simulink model "main"  (R2020b)
settings: Solver=ode23tb  StartTime=0.0  StopTime=20  FixedStep=0.0005  MaxStep=0.005  RelTol=1e-3  AbsTol=1e-3
StartFcn:
  | tic;
StopFcn:
  | Elapsed_Sim_Time = toc;
  | disp(['Elapsed Sim Time = ' num2str(Elapsed_Sim_Time)]);
model workspace (MATLAB code in the model file):
  | floor_l = 1.0900;
  | floor_d = 0.0100;
  | 
  | % PART
  | model_idx = 0;
  | model_dims = [0.06 0.06 0.06;
  |      0.02 0.05 0.07;
  |      0.04 0.04 0.10;
  |      0.05 0.05 0.05;
  |      0.10 0.08 0.08];
  | % distance between models on the conveyor belt
  | model_d = 0.12;
  | % distance to push models forwards in the -y dir (towards the box)
  | model_push = 0.2;
  | 
  | % BELT
  | belt_w = 0.1000;
  | belt_l = 1.2000;
  | belt_h = 0.0200;
  | belt_in_offset = [0 0.8000 0.0100];
  | 
  | container_belt_h = 0.02;
  | container_belt_l = 2.0;
  | container_belt_w = 0.2;
  | container_belt_offset = [-0.5050 0 -0.020];
  | 
  | belt_spd = 0.1;
  | 
  | % Model
  | cube_d = 0.06;
  | cube_z_off = belt_in_offset(3) + (container_belt_h / 2) + 0.001;
  | cube_z_offs = (model_dims(:,3) / 2) + cube_z_off;
  | 
  | % Container dimensions
  | % len, width, height are INTERNAL (Changed because most things were using internal anyway and it's 4am and we just need a working demo)
  | % Dimensions
  | container_len = 0.2;
  | container_width = 0.15;
  | container_height = 0.15;
  | container_thickness = 0.005;
  | 
  | 
  | % ????
  | cube_con_rsph = 0.003;
  | 
  | cube_con_k = 1000000;
  | cube_con_b = 1000;
  | 
  | finger_con_x = 0.01;
  | finger_con_y = 0.01;
  | finger_con_z = 5e-4;
  | finger_con_rsph = 5.0000e-04;
  | finger_con_muk = 0.05;
  | finger_con_mus = 0.07;
  | finger_con_vth = 1e-3;
  | 
  | finger_l = 0.4;
  | finger_w = 0.03;
  | finger_t = 0.01;
undefined symbols (not defined in the file): Bottom, Extr_Data_LinkHoles, Part1, Part2, Part3, Part4, Part5, point1, point2, point3, Side1, Side2, Side3, Side4, X, Y, Z
libraries: sm_lib x113, nesl_utility x35, Parts_Lib x10, Contact_Forces_Lib x6, sm_delta_robot_lib x1
(part 4 of 5)

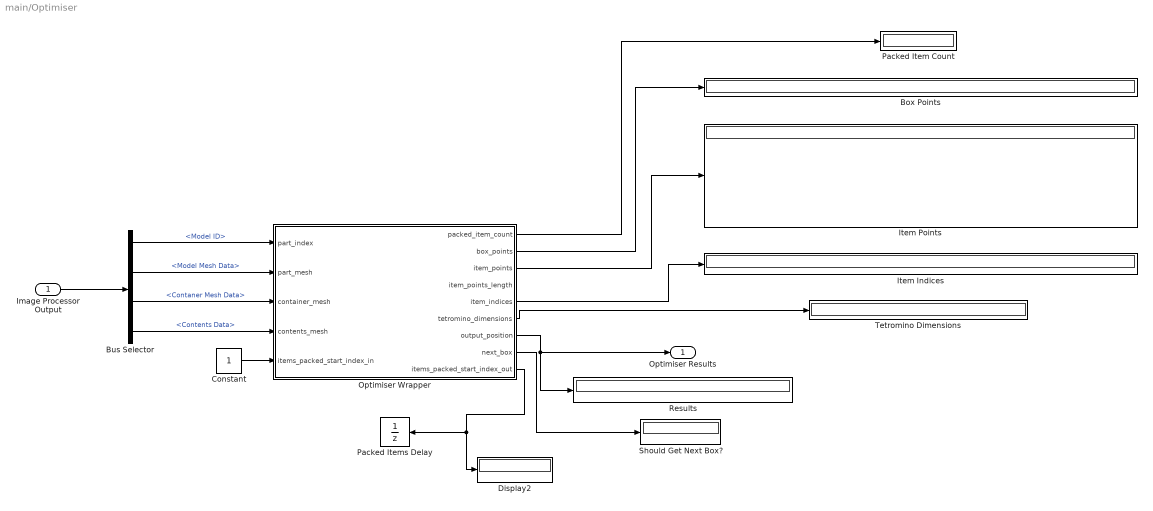
== system main/Optimiser ==
  Image Processor Output : Inport
  Box Points : Display
  Bus Selector : BusSelector  OutputSignals=Model ID,Model Mesh Data,Contaner Mesh Data,Contents Data
  Constant : Constant
  Display2 : Display
  Item Indices : Display
  Item Points : Display
  Optimiser Wrapper : MATLAB Function  TreatAsAtomicUnit=on
  Packed Item Count : Display
  Packed Items Delay : UnitDelay  InitialCondition=1  SampleTime=-1  HasFrameUpgradeWarning=on
  Results : Display
  Should Get Next Box? : Display
  Tetromino Dimensions : Display
  Optimiser Results : Outport
  wires:
  Optimiser Wrapper/8(next_box) -> Should Get Next Box?/1
  Optimiser Wrapper/9(items_packed_start_index_out) -> Packed Items Delay/1, Display2/1
  Optimiser Wrapper/2(box_points) -> Box Points/1
  Optimiser Wrapper/3(item_points) -> Item Points/1
  Optimiser Wrapper/5(item_indices) -> Item Indices/1
  Optimiser Wrapper/6(tetromino_dimensions) -> Tetromino Dimensions/1
  Image Processor Output/1 -> Bus Selector/1
  Bus Selector/1 -> Optimiser Wrapper/1(part_index)  "<Model ID>"
  Bus Selector/2 -> Optimiser Wrapper/2(part_mesh)  "<Model Mesh Data>"
  Bus Selector/3 -> Optimiser Wrapper/3(container_mesh)  "<Contaner Mesh Data>"
  Bus Selector/4 -> Optimiser Wrapper/4(contents_mesh)  "<Contents Data>"
  Optimiser Wrapper/1(packed_item_count) -> Packed Item Count/1
  Optimiser Wrapper/7(output_position) -> Optimiser Results/1, Results/1
  Constant/1 -> Optimiser Wrapper/5(items_packed_start_index_in)

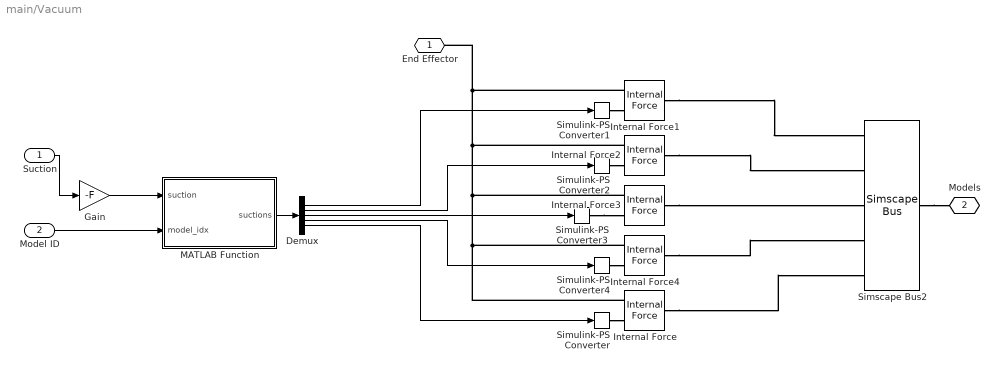
== system main/Vacuum ==
  Suction : Inport
  Model ID : Inport  Port=2
  Demux : Demux  Outputs=5
  Gain : Gain  Gain=-F
  Internal Force{,1..4} (5 alike) : sm_lib/Forces and Torques/Internal Force
      settings: SourceProductName=Multibody
  MATLAB Function : MATLAB Function  TreatAsAtomicUnit=on
  Simscape Bus2 : SimscapeBus  HierarchyStrings=Part1;Part2;Part3;Part4;Part5
  Simulink-PS Converter{,1..4} (5 alike) : nesl_utility/Simulink-PS Converter  PhysicalDomain=network_engine_domain  SubClassName=ps_input  LeftPortType=input  RightPortType=output  PseudoPeriodic=off  Frequencies=[]  NoiseDistribution=none  NoiseParameters=[]  Unit=N  AffineConversion=off  FilteringAndDerivatives=provide  SimscapeFilterOrder=1  InputFilterTimeConstant=0.001  UdotUserProvided=0
      settings: SourceProductName=Utilities
  End Effector : PMIOPort  Side=Right
  Models : PMIOPort  Port=2  Side=Right
  wires:
  Suction/1 -> Gain/1
  MATLAB Function/1(suctions) -> Demux/1
  Gain/1 -> MATLAB Function/1(suction)
  Demux/1 -> Simulink-PS Converter1/1
  Demux/2 -> Simulink-PS Converter2/1
  Demux/3 -> Simulink-PS Converter3/1
  Demux/4 -> Simulink-PS Converter4/1
  Demux/5 -> Simulink-PS Converter/1
  Model ID/1 -> MATLAB Function/2(model_idx)
  connections:
  Internal Force/RConn1 -- Simscape Bus2/LConn5
  Internal Force/LConn1 -- Internal Force4/LConn1 -- Internal Force3/LConn1 -- Internal Force2/LConn1 -- End Effector/RConn1 -- Internal Force1/LConn1
  Simulink-PS Converter/RConn1 -- Internal Force/LConn2
  Simscape Bus2/RConn1 -- Models/RConn1
  Simulink-PS Converter1/RConn1 -- Internal Force1/LConn2
  Simulink-PS Converter2/RConn1 -- Internal Force2/LConn2
  Simulink-PS Converter3/RConn1 -- Internal Force3/LConn2
  Simulink-PS Converter4/RConn1 -- Internal Force4/LConn2
  Internal Force4/RConn1 -- Simscape Bus2/LConn4
  Internal Force3/RConn1 -- Simscape Bus2/LConn3
  Internal Force2/RConn1 -- Simscape Bus2/LConn2
  Internal Force1/RConn1 -- Simscape Bus2/LConn1

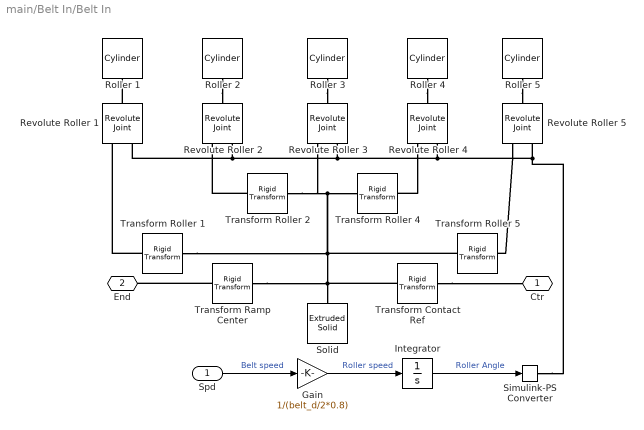
== system main/Belt In/Belt In ==
  Spd : Inport
  Gain : Gain  Gain=1/(belt_d/2*0.8)
  Integrator : Integrator
  Revolute Roller {1..5} (5 alike) : sm_lib/Joints/Revolute Joint  JointMode=Normal  SenseConstraintForce=off  SenseConstraintForceX=off  SenseConstraintForceY=off  SenseConstraintForceZ=off  SenseConstraintTorque=off  SenseConstraintTorqueX=off  SenseConstraintTorqueY=off  SenseConstraintTorqueZ=off  SenseTotalForce=off  SenseTotalForceX=off  SenseTotalForceY=off  SenseTotalForceZ=off  SenseTotalTorque=off  SenseTotalTorqueX=off  SenseTotalTorqueY=off  SenseTotalTorqueZ=off  CompositeWrenchDir=FollowerOnBase  CompositeWrenchFrame=BaseFrame  EquilibriumPosition=0  EquilibriumPositionUnits=deg  SpringStiffness=0  SpringStiffnessUnits=N*m/deg  DampingCoefficient=0  DampingCoefficientUnits=N*m/(deg/s)  TorqueActuationMode=ComputedTorque  MotionActuationMode=InputMotion  SensePosition=off  SenseVelocity=off  SenseAcceleration=off  SenseTorqueForce=off  SenseLowerLimitTorqueForce=off  SenseUpperLimitTorqueForce=off  LowerLimitSpecify=off  LowerLimitBound=-90  LowerLimitBoundUnits=deg  LowerLimitStiffness=1e4  LowerLimitStiffnessUnits=N*m/deg  LowerLimitDamping=10  LowerLimitDampingUnits=N*m/(deg/s)  LowerLimitTransitionRegionWidth=0.1  LowerLimitTransitionRegionWidthUnits=deg  UpperLimitSpecify=off  UpperLimitBound=90  UpperLimitBoundUnits=deg  UpperLimitStiffness=1e4  UpperLimitStiffnessUnits=N*m/deg  UpperLimitDamping=10  UpperLimitDampingUnits=N*m/(deg/s)  UpperLimitTransitionRegionWidth=0.1  UpperLimitTransitionRegionWidthUnits=deg  PositionTargetSpecify=off  PositionTargetPriority=High  PositionTargetValue=0  PositionTargetValueUnits=deg  VelocityTargetSpecify=off  VelocityTargetPriority=High  VelocityTargetValue=0  VelocityTargetValueUnits=deg/s
  Roller {1..5} (5 alike) : Parts_Lib/Cylinder  Tag=CustomStyle  cyl_radius=belt_d/2*0.8  cyl_length=belt_w  cyl_density=1000  cyl_color=custom  cyl_opacity=1  cyl_color_custom=roller_clr  mark_radius=[0.75 0.5]  mark_len_factor=1.01  mark_angle=60  mark_color=black  mark_opacity=1
  Simulink-PS Converter : nesl_utility/Simulink-PS Converter  PhysicalDomain=network_engine_domain  SubClassName=ps_input  LeftPortType=input  RightPortType=output  PseudoPeriodic=off  Frequencies=[]  NoiseDistribution=none  NoiseParameters=[]  Unit=1  AffineConversion=off  FilteringAndDerivatives=filter  SimscapeFilterOrder=2  InputFilterTimeConstant=0.005  UdotUserProvided=1
  Solid : sm_lib/Body Elements/Extruded Solid  GraphicAmbientColor=[0.15 0.15 0.15 1.0]  BasedOnType=Density  CenterOfMass=[0 0 0]  CenterOfMassUnits=m  GraphicDiffuseColor=[0.5 0.5 0.5]  ExportConvexHullGeometry=off  ExtrusionCrossSection=Extr_Data_LinkHoles(belt_l,belt_d,0.8*belt_d/2,5)  ExtrusionCrossSectionUnits=m  Density=1000  DensityUnits=kg/(m^3)  DoExposeReferenceFrame=on  GraphicEmissiveColor=[0.0 0.0 0.0 1.0]  ExportEntireGeometry=off  ExtrusionLength=belt_w  ExtrusionLengthUnits=m  ExtrusionType=General  SerializedFrames=<Frames/>  MarkerShape=Sphere  MarkerSize=10  GraphicType=FromGeometry  InertiaType=CalculateFromGeometry  Mass=1  MassUnits=kg  MomentsOfInertia=[1 1 1]  MomentsOfInertiaUnits=kg*m^2  PolygonNumSides=3  GraphicOpacity=1.0  PolygonOuterRadius=1  PolygonOuterRadiusUnits=m  ProductsOfInertia=[0 0 0]  ProductsOfInertiaUnits=kg*m^2  GraphicShininess=75  GraphicSpecularColor=[0.5 0.5 0.5 1.0]  GraphicVisPropType=SimpleVisualProperties
  Transform Contact Ref : sm_lib/Frames and Transforms/Rigid Transform  TranslationMethod=None  TranslationStandardOffset=3/2  TranslationLengthUnit=m  TranslationStandardAxis=+X  TranslationCartesianOffset=[0 0 0]  TranslationROffset=0  TranslationROffsetUnits=m  TranslationZOffset=0  TranslationZOffsetUnits=m  TranslationThetaOffset=0  TranslationThetaOffsetUnits=deg  RotationMethod=RotationSequence  RotationAngleUnits=deg  RotationStandardAxis=+Z  RotationAngle=0  RotationArbitraryAxis=[0 0 1]  FollAlignAxisA=+X  BaseAlignAxisA=+Y  FollAlignAxisB=+Y  BaseAlignAxisB=+Z  RotationSequenceAxes=FollowerAxes  RotationSequence=XYZ  RotationSequenceAngles=[-90 0 0]  RotationSequenceAnglesUnits=deg  RotationMatrix=[1 0 0; 0 1 0; 0 0 1]
  Transform Ramp Center : sm_lib/Frames and Transforms/Rigid Transform  TranslationMethod=StandardAxis  TranslationStandardOffset=belt_l/2  TranslationLengthUnit=m  TranslationStandardAxis=-X  TranslationCartesianOffset=[0 0 0]  TranslationROffset=0  TranslationROffsetUnits=m  TranslationZOffset=0  TranslationZOffsetUnits=m  TranslationThetaOffset=0  TranslationThetaOffsetUnits=deg  RotationMethod=None  RotationAngleUnits=deg  RotationStandardAxis=+Z  RotationAngle=0  RotationArbitraryAxis=[0 0 1]  FollAlignAxisA=+X  BaseAlignAxisA=+Y  FollAlignAxisB=+Y  BaseAlignAxisB=+Z  RotationSequenceAxes=FollowerAxes  RotationSequence=XYX  RotationSequenceAngles=[0 0 0]  RotationSequenceAnglesUnits=deg  RotationMatrix=[1 0 0; 0 1 0; 0 0 1]
  Transform Roller 1 : sm_lib/Frames and Transforms/Rigid Transform  TranslationMethod=StandardAxis  TranslationStandardOffset=belt_l/2  TranslationLengthUnit=m  TranslationStandardAxis=-X  TranslationCartesianOffset=[0 0 0]  TranslationROffset=0  TranslationROffsetUnits=m  TranslationZOffset=0  TranslationZOffsetUnits=m  TranslationThetaOffset=0  TranslationThetaOffsetUnits=deg  RotationMethod=None  RotationAngleUnits=deg  RotationStandardAxis=+Z  RotationAngle=0  RotationArbitraryAxis=[0 0 1]  FollAlignAxisA=+X  BaseAlignAxisA=+Y  FollAlignAxisB=+Y  BaseAlignAxisB=+Z  RotationSequenceAxes=FollowerAxes  RotationSequence=XYX  RotationSequenceAngles=[0 0 0]  RotationSequenceAnglesUnits=deg  RotationMatrix=[1 0 0; 0 1 0; 0 0 1]
  Transform Roller 2 : sm_lib/Frames and Transforms/Rigid Transform  TranslationMethod=StandardAxis  TranslationStandardOffset=belt_l/4  TranslationLengthUnit=m  TranslationStandardAxis=-X  TranslationCartesianOffset=[0 0 0]  TranslationROffset=0  TranslationROffsetUnits=m  TranslationZOffset=0  TranslationZOffsetUnits=m  TranslationThetaOffset=0  TranslationThetaOffsetUnits=deg  RotationMethod=None  RotationAngleUnits=deg  RotationStandardAxis=+Z  RotationAngle=0  RotationArbitraryAxis=[0 0 1]  FollAlignAxisA=+X  BaseAlignAxisA=+Y  FollAlignAxisB=+Y  BaseAlignAxisB=+Z  RotationSequenceAxes=FollowerAxes  RotationSequence=XYX  RotationSequenceAngles=[0 0 0]  RotationSequenceAnglesUnits=deg  RotationMatrix=[1 0 0; 0 1 0; 0 0 1]
  Transform Roller 4 : sm_lib/Frames and Transforms/Rigid Transform  TranslationMethod=StandardAxis  TranslationStandardOffset=belt_l/4  TranslationLengthUnit=m  TranslationStandardAxis=+X  TranslationCartesianOffset=[0 0 0]  TranslationROffset=0  TranslationROffsetUnits=m  TranslationZOffset=0  TranslationZOffsetUnits=m  TranslationThetaOffset=0  TranslationThetaOffsetUnits=deg  RotationMethod=None  RotationAngleUnits=deg  RotationStandardAxis=+Z  RotationAngle=0  RotationArbitraryAxis=[0 0 1]  FollAlignAxisA=+X  BaseAlignAxisA=+Y  FollAlignAxisB=+Y  BaseAlignAxisB=+Z  RotationSequenceAxes=FollowerAxes  RotationSequence=XYX  RotationSequenceAngles=[0 0 0]  RotationSequenceAnglesUnits=deg  RotationMatrix=[1 0 0; 0 1 0; 0 0 1]
  Transform Roller 5 : sm_lib/Frames and Transforms/Rigid Transform  TranslationMethod=StandardAxis  TranslationStandardOffset=belt_l/2  TranslationLengthUnit=m  TranslationStandardAxis=+X  TranslationCartesianOffset=[0 0 0]  TranslationROffset=0  TranslationROffsetUnits=m  TranslationZOffset=0  TranslationZOffsetUnits=m  TranslationThetaOffset=0  TranslationThetaOffsetUnits=deg  RotationMethod=None  RotationAngleUnits=deg  RotationStandardAxis=+Z  RotationAngle=0  RotationArbitraryAxis=[0 0 1]  FollAlignAxisA=+X  BaseAlignAxisA=+Y  FollAlignAxisB=+Y  BaseAlignAxisB=+Z  RotationSequenceAxes=FollowerAxes  RotationSequence=XYX  RotationSequenceAngles=[0 0 0]  RotationSequenceAnglesUnits=deg  RotationMatrix=[1 0 0; 0 1 0; 0 0 1]
  Ctr : PMIOPort  Side=Right
  End : PMIOPort  Port=2  Side=Left
  wires:
  Integrator/1 -> Simulink-PS Converter/1  "Roller Angle"
  Gain/1 -> Integrator/1  "Roller speed"
  Spd/1 -> Gain/1  "Belt speed"
  connections:
  Revolute Roller 5/LConn2 -- Revolute Roller 4/LConn2 -- Revolute Roller 3/LConn2 -- Revolute Roller 2/LConn2 -- Revolute Roller 1/LConn2 -- Simulink-PS Converter/RConn1
  Roller 5/LConn1 -- Revolute Roller 5/RConn1
  Roller 4/LConn1 -- Revolute Roller 4/RConn1
  Roller 3/LConn1 -- Revolute Roller 3/RConn1
  Roller 2/LConn1 -- Revolute Roller 2/RConn1
  Transform Roller 1/RConn1 -- Revolute Roller 1/LConn1
  Revolute Roller 5/LConn1 -- Transform Roller 5/RConn1
  Revolute Roller 4/LConn1 -- Transform Roller 4/RConn1
  Transform Roller 2/RConn1 -- Revolute Roller 2/LConn1
  Revolute Roller 1/RConn1 -- Roller 1/LConn1
  Transform Ramp Center/LConn1 -- End/RConn1
  Transform Contact Ref/RConn1 -- Transform Ramp Center/RConn1 -- Transform Roller 5/LConn1 -- Transform Roller 1/LConn1 -- Transform Roller 4/LConn1 -- Transform Roller 2/LConn1 -- Revolute Roller 3/LConn1 -- Solid/RConn1
  Transform Contact Ref/LConn1 -- Ctr/RConn1

== system main/Belt In/Create Bus Belt In1 ==
  On : Inport
  Belt Speed : Gain  Gain=belt_spd
  Bus Creator : BusCreator  Inputs=3
  Constant : Constant
  Constant1 : Constant  Value=0
  bus : Outport  VectorParamsAs1DForOutWhenUnconnected=off
  wires:
  Constant1/1 -> Bus Creator/3  "vy"
  On/1 -> Belt Speed/1
  Constant/1 -> Bus Creator/1  "Enable"
  Bus Creator/1 -> bus/1
  Belt Speed/1 -> Bus Creator/2  "vx"

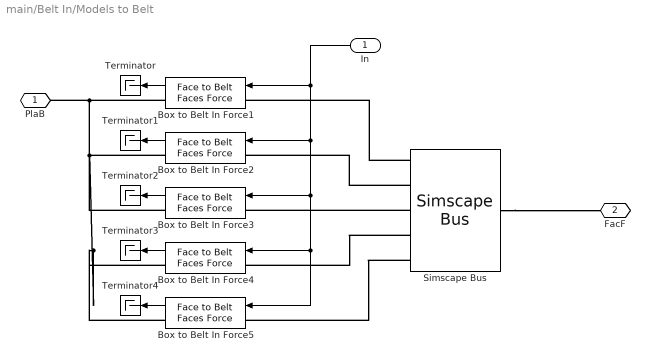
== system main/Belt In/Models to Belt ==
  In : Inport
  Box to Belt In Force1 : Contact_Forces_Lib/3D/Composite Forces/Face to Belt Faces Force  PlaB_x=belt_l  PlaB_y=belt_w  PlaB_z=belt_h/2  FacF_x=model_dims(1, 1)  FacF_y=model_dims(1, 2)  FacF_z=model_dims(1, 3)/2  FacF_rSph=cube_con_rsph  force_law_pla2pla=Linear  k_contact_pla2pla=stff  b_contact_pla2pla=dmp  pen_full_damp_F_pla2pla=1e-4  pen_exponent_pla2pla=1  friction_law_pla2pla=Stick-Slip Continuous  mu_kinetic_pla2pla=0.5  mu_static_pla2pla=0.7  v_thr_pla2pla=0.001  vis_on_pla2pla=off  vis_opc_en_box2box=0  vis_len_plaLz=0.0005  vis_clr=[0.9 0.2 0.2]  vis_opc=0.7
      settings: SourceProductName=Simscape Multibody Contact Forces Library
  Box to Belt In Force2 : Contact_Forces_Lib/3D/Composite Forces/Face to Belt Faces Force  PlaB_x=belt_l  PlaB_y=belt_w  PlaB_z=belt_h/2  FacF_x=model_dims(2, 1)  FacF_y=model_dims(2, 2)  FacF_z=model_dims(2, 3)/2  FacF_rSph=cube_con_rsph  force_law_pla2pla=Linear  k_contact_pla2pla=stff  b_contact_pla2pla=dmp  pen_full_damp_F_pla2pla=1e-4  pen_exponent_pla2pla=1  friction_law_pla2pla=Stick-Slip Continuous  mu_kinetic_pla2pla=0.5  mu_static_pla2pla=0.7  v_thr_pla2pla=0.001  vis_on_pla2pla=off  vis_opc_en_box2box=0  vis_len_plaLz=0.0005  vis_clr=[0.9 0.2 0.2]  vis_opc=0.7
      settings: SourceProductName=Simscape Multibody Contact Forces Library
  Box to Belt In Force3 : Contact_Forces_Lib/3D/Composite Forces/Face to Belt Faces Force  PlaB_x=belt_l  PlaB_y=belt_w  PlaB_z=belt_h/2  FacF_x=model_dims(3, 1)  FacF_y=model_dims(3, 2)  FacF_z=model_dims(3, 3)/2  FacF_rSph=cube_con_rsph  force_law_pla2pla=Linear  k_contact_pla2pla=stff  b_contact_pla2pla=dmp  pen_full_damp_F_pla2pla=1e-4  pen_exponent_pla2pla=1  friction_law_pla2pla=Stick-Slip Continuous  mu_kinetic_pla2pla=0.5  mu_static_pla2pla=0.7  v_thr_pla2pla=0.001  vis_on_pla2pla=off  vis_opc_en_box2box=0  vis_len_plaLz=0.0005  vis_clr=[0.9 0.2 0.2]  vis_opc=0.7
      settings: SourceProductName=Simscape Multibody Contact Forces Library
  Box to Belt In Force4 : Contact_Forces_Lib/3D/Composite Forces/Face to Belt Faces Force  PlaB_x=belt_l  PlaB_y=belt_w  PlaB_z=belt_h/2  FacF_x=model_dims(4, 1)  FacF_y=model_dims(4, 2)  FacF_z=model_dims(4, 3)/2  FacF_rSph=cube_con_rsph  force_law_pla2pla=Linear  k_contact_pla2pla=stff  b_contact_pla2pla=dmp  pen_full_damp_F_pla2pla=1e-4  pen_exponent_pla2pla=1  friction_law_pla2pla=Stick-Slip Continuous  mu_kinetic_pla2pla=0.5  mu_static_pla2pla=0.7  v_thr_pla2pla=0.001  vis_on_pla2pla=off  vis_opc_en_box2box=0  vis_len_plaLz=0.0005  vis_clr=[0.9 0.2 0.2]  vis_opc=0.7
      settings: SourceProductName=Simscape Multibody Contact Forces Library
  Box to Belt In Force5 : Contact_Forces_Lib/3D/Composite Forces/Face to Belt Faces Force  PlaB_x=belt_l  PlaB_y=belt_w  PlaB_z=belt_h/2  FacF_x=model_dims(5, 1)  FacF_y=model_dims(5, 2)  FacF_z=model_dims(5, 3)/2  FacF_rSph=cube_con_rsph  force_law_pla2pla=Linear  k_contact_pla2pla=stff  b_contact_pla2pla=dmp  pen_full_damp_F_pla2pla=1e-4  pen_exponent_pla2pla=1  friction_law_pla2pla=Stick-Slip Continuous  mu_kinetic_pla2pla=0.5  mu_static_pla2pla=0.7  v_thr_pla2pla=0.001  vis_on_pla2pla=off  vis_opc_en_box2box=0  vis_len_plaLz=0.0005  vis_clr=[0.9 0.2 0.2]  vis_opc=0.7
      settings: SourceProductName=Simscape Multibody Contact Forces Library
  Simscape Bus : SimscapeBus  HierarchyStrings=Part1;Part2;Part3;Part4;Part5
  Terminator{,1..4} (5 alike) : Terminator
  PlaB : PMIOPort  Side=Right
  FacF : PMIOPort  Port=2  Side=Left
  wires:
  Box to Belt In Force1/1 -> Terminator/1
  In/1 -> Box to Belt In Force1/1, Box to Belt In Force5/1, Box to Belt In Force4/1, Box to Belt In Force3/1, Box to Belt In Force2/1
  Box to Belt In Force2/1 -> Terminator1/1
  Box to Belt In Force5/1 -> Terminator4/1
  Box to Belt In Force4/1 -> Terminator3/1
  Box to Belt In Force3/1 -> Terminator2/1
  connections:
  Box to Belt In Force1/RConn1 -- Box to Belt In Force5/RConn1 -- Box to Belt In Force4/RConn1 -- Box to Belt In Force3/RConn1 -- Box to Belt In Force2/RConn1 -- PlaB/RConn1
  Simscape Bus/RConn1 -- FacF/RConn1
  Simscape Bus/LConn1 -- Box to Belt In Force1/LConn1
  Simscape Bus/LConn2 -- Box to Belt In Force2/LConn1
  Simscape Bus/LConn3 -- Box to Belt In Force3/LConn1
  Simscape Bus/LConn4 -- Box to Belt In Force4/LConn1
  Simscape Bus/LConn5 -- Box to Belt In Force5/LConn1

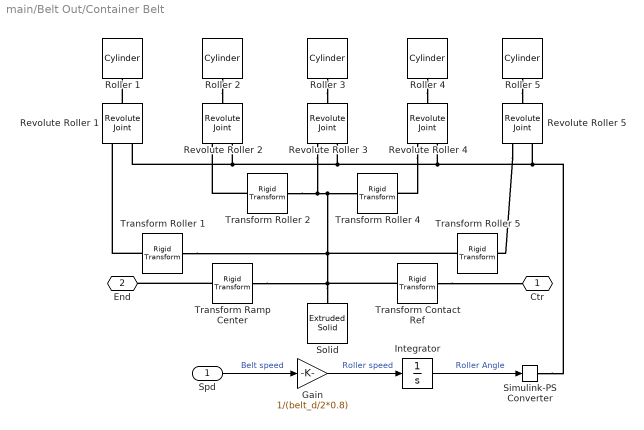
== system main/Belt Out/Container Belt ==
  Spd : Inport
  Gain : Gain  Gain=1/(belt_d/2*0.8)
  Integrator : Integrator
  Revolute Roller {1..5} (5 alike) : sm_lib/Joints/Revolute Joint  JointMode=Normal  SenseConstraintForce=off  SenseConstraintForceX=off  SenseConstraintForceY=off  SenseConstraintForceZ=off  SenseConstraintTorque=off  SenseConstraintTorqueX=off  SenseConstraintTorqueY=off  SenseConstraintTorqueZ=off  SenseTotalForce=off  SenseTotalForceX=off  SenseTotalForceY=off  SenseTotalForceZ=off  SenseTotalTorque=off  SenseTotalTorqueX=off  SenseTotalTorqueY=off  SenseTotalTorqueZ=off  CompositeWrenchDir=FollowerOnBase  CompositeWrenchFrame=BaseFrame  EquilibriumPosition=0  EquilibriumPositionUnits=deg  SpringStiffness=0  SpringStiffnessUnits=N*m/deg  DampingCoefficient=0  DampingCoefficientUnits=N*m/(deg/s)  TorqueActuationMode=ComputedTorque  MotionActuationMode=InputMotion  SensePosition=off  SenseVelocity=off  SenseAcceleration=off  SenseTorqueForce=off  SenseLowerLimitTorqueForce=off  SenseUpperLimitTorqueForce=off  LowerLimitSpecify=off  LowerLimitBound=-90  LowerLimitBoundUnits=deg  LowerLimitStiffness=1e4  LowerLimitStiffnessUnits=N*m/deg  LowerLimitDamping=10  LowerLimitDampingUnits=N*m/(deg/s)  LowerLimitTransitionRegionWidth=0.1  LowerLimitTransitionRegionWidthUnits=deg  UpperLimitSpecify=off  UpperLimitBound=90  UpperLimitBoundUnits=deg  UpperLimitStiffness=1e4  UpperLimitStiffnessUnits=N*m/deg  UpperLimitDamping=10  UpperLimitDampingUnits=N*m/(deg/s)  UpperLimitTransitionRegionWidth=0.1  UpperLimitTransitionRegionWidthUnits=deg  PositionTargetSpecify=off  PositionTargetPriority=High  PositionTargetValue=0  PositionTargetValueUnits=deg  VelocityTargetSpecify=off  VelocityTargetPriority=High  VelocityTargetValue=0  VelocityTargetValueUnits=deg/s
  Roller {1..5} (5 alike) : Parts_Lib/Cylinder  Tag=CustomStyle  cyl_radius=belt_d/2*0.8  cyl_length=belt_w  cyl_density=1000  cyl_color=custom  cyl_opacity=1  cyl_color_custom=roller_clr  mark_radius=[0.75 0.5]  mark_len_factor=1.01  mark_angle=60  mark_color=black  mark_opacity=1
  Simulink-PS Converter : nesl_utility/Simulink-PS Converter  PhysicalDomain=network_engine_domain  SubClassName=ps_input  LeftPortType=input  RightPortType=output  PseudoPeriodic=off  Frequencies=[]  NoiseDistribution=none  NoiseParameters=[]  Unit=1  AffineConversion=off  FilteringAndDerivatives=filter  SimscapeFilterOrder=2  InputFilterTimeConstant=0.005  UdotUserProvided=1
  Solid : sm_lib/Body Elements/Extruded Solid  GraphicAmbientColor=[0.15 0.15 0.15 1.0]  BasedOnType=Density  CenterOfMass=[0 0 0]  CenterOfMassUnits=m  GraphicDiffuseColor=[0.5 0.5 0.5]  ExportConvexHullGeometry=off  ExtrusionCrossSection=Extr_Data_LinkHoles(belt_l,belt_d,0.8*belt_d/2,5)  ExtrusionCrossSectionUnits=m  Density=1000  DensityUnits=kg/(m^3)  DoExposeReferenceFrame=on  GraphicEmissiveColor=[0.0 0.0 0.0 1.0]  ExportEntireGeometry=off  ExtrusionLength=belt_w  ExtrusionLengthUnits=m  ExtrusionType=General  SerializedFrames=<Frames/>  MarkerShape=Sphere  MarkerSize=10  GraphicType=FromGeometry  InertiaType=CalculateFromGeometry  Mass=1  MassUnits=kg  MomentsOfInertia=[1 1 1]  MomentsOfInertiaUnits=kg*m^2  PolygonNumSides=3  GraphicOpacity=1.0  PolygonOuterRadius=1  PolygonOuterRadiusUnits=m  ProductsOfInertia=[0 0 0]  ProductsOfInertiaUnits=kg*m^2  GraphicShininess=75  GraphicSpecularColor=[0.5 0.5 0.5 1.0]  GraphicVisPropType=SimpleVisualProperties
  Transform Contact Ref : sm_lib/Frames and Transforms/Rigid Transform  TranslationMethod=None  TranslationStandardOffset=3/2  TranslationLengthUnit=m  TranslationStandardAxis=+X  TranslationCartesianOffset=[0 0 0]  TranslationROffset=0  TranslationROffsetUnits=m  TranslationZOffset=0  TranslationZOffsetUnits=m  TranslationThetaOffset=0  TranslationThetaOffsetUnits=deg  RotationMethod=RotationSequence  RotationAngleUnits=deg  RotationStandardAxis=+Z  RotationAngle=0  RotationArbitraryAxis=[0 0 1]  FollAlignAxisA=+X  BaseAlignAxisA=+Y  FollAlignAxisB=+Y  BaseAlignAxisB=+Z  RotationSequenceAxes=FollowerAxes  RotationSequence=XYZ  RotationSequenceAngles=[-90 0 0]  RotationSequenceAnglesUnits=deg  RotationMatrix=[1 0 0; 0 1 0; 0 0 1]
  Transform Ramp Center : sm_lib/Frames and Transforms/Rigid Transform  TranslationMethod=StandardAxis  TranslationStandardOffset=belt_l/2  TranslationLengthUnit=m  TranslationStandardAxis=-X  TranslationCartesianOffset=[0 0 0]  TranslationROffset=0  TranslationROffsetUnits=m  TranslationZOffset=0  TranslationZOffsetUnits=m  TranslationThetaOffset=0  TranslationThetaOffsetUnits=deg  RotationMethod=None  RotationAngleUnits=deg  RotationStandardAxis=+Z  RotationAngle=0  RotationArbitraryAxis=[0 0 1]  FollAlignAxisA=+X  BaseAlignAxisA=+Y  FollAlignAxisB=+Y  BaseAlignAxisB=+Z  RotationSequenceAxes=FollowerAxes  RotationSequence=XYX  RotationSequenceAngles=[0 0 0]  RotationSequenceAnglesUnits=deg  RotationMatrix=[1 0 0; 0 1 0; 0 0 1]
  Transform Roller 1 : sm_lib/Frames and Transforms/Rigid Transform  TranslationMethod=StandardAxis  TranslationStandardOffset=belt_l/2  TranslationLengthUnit=m  TranslationStandardAxis=-X  TranslationCartesianOffset=[0 0 0]  TranslationROffset=0  TranslationROffsetUnits=m  TranslationZOffset=0  TranslationZOffsetUnits=m  TranslationThetaOffset=0  TranslationThetaOffsetUnits=deg  RotationMethod=None  RotationAngleUnits=deg  RotationStandardAxis=+Z  RotationAngle=0  RotationArbitraryAxis=[0 0 1]  FollAlignAxisA=+X  BaseAlignAxisA=+Y  FollAlignAxisB=+Y  BaseAlignAxisB=+Z  RotationSequenceAxes=FollowerAxes  RotationSequence=XYX  RotationSequenceAngles=[0 0 0]  RotationSequenceAnglesUnits=deg  RotationMatrix=[1 0 0; 0 1 0; 0 0 1]
  Transform Roller 2 : sm_lib/Frames and Transforms/Rigid Transform  TranslationMethod=StandardAxis  TranslationStandardOffset=belt_l/4  TranslationLengthUnit=m  TranslationStandardAxis=-X  TranslationCartesianOffset=[0 0 0]  TranslationROffset=0  TranslationROffsetUnits=m  TranslationZOffset=0  TranslationZOffsetUnits=m  TranslationThetaOffset=0  TranslationThetaOffsetUnits=deg  RotationMethod=None  RotationAngleUnits=deg  RotationStandardAxis=+Z  RotationAngle=0  RotationArbitraryAxis=[0 0 1]  FollAlignAxisA=+X  BaseAlignAxisA=+Y  FollAlignAxisB=+Y  BaseAlignAxisB=+Z  RotationSequenceAxes=FollowerAxes  RotationSequence=XYX  RotationSequenceAngles=[0 0 0]  RotationSequenceAnglesUnits=deg  RotationMatrix=[1 0 0; 0 1 0; 0 0 1]
  Transform Roller 4 : sm_lib/Frames and Transforms/Rigid Transform  TranslationMethod=StandardAxis  TranslationStandardOffset=belt_l/4  TranslationLengthUnit=m  TranslationStandardAxis=+X  TranslationCartesianOffset=[0 0 0]  TranslationROffset=0  TranslationROffsetUnits=m  TranslationZOffset=0  TranslationZOffsetUnits=m  TranslationThetaOffset=0  TranslationThetaOffsetUnits=deg  RotationMethod=None  RotationAngleUnits=deg  RotationStandardAxis=+Z  RotationAngle=0  RotationArbitraryAxis=[0 0 1]  FollAlignAxisA=+X  BaseAlignAxisA=+Y  FollAlignAxisB=+Y  BaseAlignAxisB=+Z  RotationSequenceAxes=FollowerAxes  RotationSequence=XYX  RotationSequenceAngles=[0 0 0]  RotationSequenceAnglesUnits=deg  RotationMatrix=[1 0 0; 0 1 0; 0 0 1]
  Transform Roller 5 : sm_lib/Frames and Transforms/Rigid Transform  TranslationMethod=StandardAxis  TranslationStandardOffset=belt_l/2  TranslationLengthUnit=m  TranslationStandardAxis=+X  TranslationCartesianOffset=[0 0 0]  TranslationROffset=0  TranslationROffsetUnits=m  TranslationZOffset=0  TranslationZOffsetUnits=m  TranslationThetaOffset=0  TranslationThetaOffsetUnits=deg  RotationMethod=None  RotationAngleUnits=deg  RotationStandardAxis=+Z  RotationAngle=0  RotationArbitraryAxis=[0 0 1]  FollAlignAxisA=+X  BaseAlignAxisA=+Y  FollAlignAxisB=+Y  BaseAlignAxisB=+Z  RotationSequenceAxes=FollowerAxes  RotationSequence=XYX  RotationSequenceAngles=[0 0 0]  RotationSequenceAnglesUnits=deg  RotationMatrix=[1 0 0; 0 1 0; 0 0 1]
  Ctr : PMIOPort  Side=Right
  End : PMIOPort  Port=2  Side=Left
  wires:
  Spd/1 -> Gain/1  "Belt speed"
  Gain/1 -> Integrator/1  "Roller speed"
  Integrator/1 -> Simulink-PS Converter/1  "Roller Angle"
  connections:
  Transform Contact Ref/LConn1 -- Ctr/RConn1
  Solid/RConn1 -- Revolute Roller 3/LConn1 -- Transform Roller 2/LConn1 -- Transform Roller 4/LConn1 -- Transform Roller 1/LConn1 -- Transform Roller 5/LConn1 -- Transform Ramp Center/RConn1 -- Transform Contact Ref/RConn1
  Transform Ramp Center/LConn1 -- End/RConn1
  Revolute Roller 1/RConn1 -- Roller 1/LConn1
  Transform Roller 2/RConn1 -- Revolute Roller 2/LConn1
  Revolute Roller 4/LConn1 -- Transform Roller 4/RConn1
  Revolute Roller 5/LConn1 -- Transform Roller 5/RConn1
  Transform Roller 1/RConn1 -- Revolute Roller 1/LConn1
  Roller 2/LConn1 -- Revolute Roller 2/RConn1
  Roller 3/LConn1 -- Revolute Roller 3/RConn1
  Roller 4/LConn1 -- Revolute Roller 4/RConn1
  Roller 5/LConn1 -- Revolute Roller 5/RConn1
  Simulink-PS Converter/RConn1 -- Revolute Roller 1/LConn2 -- Revolute Roller 2/LConn2 -- Revolute Roller 3/LConn2 -- Revolute Roller 4/LConn2 -- Revolute Roller 5/LConn2

== system main/Belt Out/Create Bus Belt Out ==
  On : Inport
  Belt Speed : Gain  Gain=belt_spd
  Bus Creator1 : BusCreator  Inputs=3
  Constant2 : Constant  Value=0
  Constant3 : Constant
  bus : Outport  VectorParamsAs1DForOutWhenUnconnected=off
  wires:
  On/1 -> Belt Speed/1
  Constant2/1 -> Bus Creator1/3  "vy"
  Bus Creator1/1 -> bus/1
  Constant3/1 -> Bus Creator1/1  "Enable"
  Belt Speed/1 -> Bus Creator1/2  "vx"

== system main/Contacts Models Container/Contacts Model-Container1 ==
  Simscape Bus : SimscapeBus  HierarchyStrings=Side1;Side2;Side3;Side4;Bottom
  Spatial Contact Force{1..3,7} (4 alike) : sm_lib/Forces and Torques/Spatial Contact Force  CoefficientOfDynamicFriction=muk  CoefficientOfStaticFriction=mus  NormalDamping=b  NormalDampingUnits=N/(m/s)  NormalStiffness=k  NormalStiffnessUnits=N/m  FrictionalCriticalVelocity=1e-3  FrictionalCriticalVelocityUnits=m/s  ZeroCrossDetectContactStartAndEnd=off  SenseFrictionalForceMagnitude=off  SenseNormalForceMagnitude=off  SenseSeparationDistance=off  NormalTransitionRegionWidth=1e-4  NormalTransitionRegionWidthUnits=m  FrictionType=SmoothStickSlip
      settings: SourceProductName=Multibody
  Spatial Contact Force4 : sm_lib/Forces and Torques/Spatial Contact Force  CoefficientOfDynamicFriction=muk  CoefficientOfStaticFriction=mus  NormalDamping=b  NormalDampingUnits=N/(m/s)  NormalStiffness=k  NormalStiffnessUnits=N/m  FrictionalCriticalVelocity=1e-3  FrictionalCriticalVelocityUnits=m/s  ZeroCrossDetectContactStartAndEnd=on  SenseFrictionalForceMagnitude=off  SenseNormalForceMagnitude=off  SenseSeparationDistance=off  NormalTransitionRegionWidth=1e-5  NormalTransitionRegionWidthUnits=m  FrictionType=SmoothStickSlip
      settings: SourceProductName=Multibody
  Container : PMIOPort  Side=Left
  Part : PMIOPort  Port=2  Side=Right
  connections:
  Spatial Contact Force4/RConn1 -- Spatial Contact Force3/RConn1 -- Part/RConn1 -- Spatial Contact Force2/RConn1 -- Spatial Contact Force1/RConn1 -- Spatial Contact Force7/RConn1
  Simscape Bus/RConn1 -- Container/RConn1
  Simscape Bus/LConn1 -- Spatial Contact Force7/LConn1
  Simscape Bus/LConn2 -- Spatial Contact Force1/LConn1
  Simscape Bus/LConn3 -- Spatial Contact Force2/LConn1
  Simscape Bus/LConn4 -- Spatial Contact Force3/LConn1
  Simscape Bus/LConn5 -- Spatial Contact Force4/LConn1

== system main/Contacts Models Container/Contacts Model-Container2 ==
  Simscape Bus : SimscapeBus  HierarchyStrings=Side1;Side2;Side3;Side4;Bottom
  Spatial Contact Force{1..3,7} (4 alike) : sm_lib/Forces and Torques/Spatial Contact Force  CoefficientOfDynamicFriction=muk  CoefficientOfStaticFriction=mus  NormalDamping=b  NormalDampingUnits=N/(m/s)  NormalStiffness=k  NormalStiffnessUnits=N/m  FrictionalCriticalVelocity=1e-3  FrictionalCriticalVelocityUnits=m/s  ZeroCrossDetectContactStartAndEnd=off  SenseFrictionalForceMagnitude=off  SenseNormalForceMagnitude=off  SenseSeparationDistance=off  NormalTransitionRegionWidth=1e-4  NormalTransitionRegionWidthUnits=m  FrictionType=SmoothStickSlip
      settings: SourceProductName=Multibody
  Spatial Contact Force4 : sm_lib/Forces and Torques/Spatial Contact Force  CoefficientOfDynamicFriction=muk  CoefficientOfStaticFriction=mus  NormalDamping=b  NormalDampingUnits=N/(m/s)  NormalStiffness=k  NormalStiffnessUnits=N/m  FrictionalCriticalVelocity=1e-3  FrictionalCriticalVelocityUnits=m/s  ZeroCrossDetectContactStartAndEnd=on  SenseFrictionalForceMagnitude=off  SenseNormalForceMagnitude=off  SenseSeparationDistance=off  NormalTransitionRegionWidth=1e-5  NormalTransitionRegionWidthUnits=m  FrictionType=SmoothStickSlip
      settings: SourceProductName=Multibody
  Container : PMIOPort  Side=Left
  Part : PMIOPort  Port=2  Side=Right
  connections:
  Spatial Contact Force4/RConn1 -- Spatial Contact Force3/RConn1 -- Part/RConn1 -- Spatial Contact Force2/RConn1 -- Spatial Contact Force1/RConn1 -- Spatial Contact Force7/RConn1
  Simscape Bus/RConn1 -- Container/RConn1
  Simscape Bus/LConn1 -- Spatial Contact Force7/LConn1
  Simscape Bus/LConn2 -- Spatial Contact Force1/LConn1
  Simscape Bus/LConn3 -- Spatial Contact Force2/LConn1
  Simscape Bus/LConn4 -- Spatial Contact Force3/LConn1
  Simscape Bus/LConn5 -- Spatial Contact Force4/LConn1

== system main/Contacts Models Container/Contacts Model-Container3 ==
  Simscape Bus : SimscapeBus  HierarchyStrings=Side1;Side2;Side3;Side4;Bottom
  Spatial Contact Force{1..3,7} (4 alike) : sm_lib/Forces and Torques/Spatial Contact Force  CoefficientOfDynamicFriction=muk  CoefficientOfStaticFriction=mus  NormalDamping=b  NormalDampingUnits=N/(m/s)  NormalStiffness=k  NormalStiffnessUnits=N/m  FrictionalCriticalVelocity=1e-3  FrictionalCriticalVelocityUnits=m/s  ZeroCrossDetectContactStartAndEnd=off  SenseFrictionalForceMagnitude=off  SenseNormalForceMagnitude=off  SenseSeparationDistance=off  NormalTransitionRegionWidth=1e-4  NormalTransitionRegionWidthUnits=m  FrictionType=SmoothStickSlip
      settings: SourceProductName=Multibody
  Spatial Contact Force4 : sm_lib/Forces and Torques/Spatial Contact Force  CoefficientOfDynamicFriction=muk  CoefficientOfStaticFriction=mus  NormalDamping=b  NormalDampingUnits=N/(m/s)  NormalStiffness=k  NormalStiffnessUnits=N/m  FrictionalCriticalVelocity=1e-3  FrictionalCriticalVelocityUnits=m/s  ZeroCrossDetectContactStartAndEnd=on  SenseFrictionalForceMagnitude=off  SenseNormalForceMagnitude=off  SenseSeparationDistance=off  NormalTransitionRegionWidth=1e-5  NormalTransitionRegionWidthUnits=m  FrictionType=SmoothStickSlip
      settings: SourceProductName=Multibody
  Container : PMIOPort  Side=Left
  Part : PMIOPort  Port=2  Side=Right
  connections:
  Spatial Contact Force4/RConn1 -- Spatial Contact Force3/RConn1 -- Part/RConn1 -- Spatial Contact Force2/RConn1 -- Spatial Contact Force1/RConn1 -- Spatial Contact Force7/RConn1
  Simscape Bus/RConn1 -- Container/RConn1
  Simscape Bus/LConn1 -- Spatial Contact Force7/LConn1
  Simscape Bus/LConn2 -- Spatial Contact Force1/LConn1
  Simscape Bus/LConn3 -- Spatial Contact Force2/LConn1
  Simscape Bus/LConn4 -- Spatial Contact Force3/LConn1
  Simscape Bus/LConn5 -- Spatial Contact Force4/LConn1

== system main/Contacts Models Container/Contacts Model-Container4 ==
  Simscape Bus : SimscapeBus  HierarchyStrings=Side1;Side2;Side3;Side4;Bottom
  Spatial Contact Force{1..3,7} (4 alike) : sm_lib/Forces and Torques/Spatial Contact Force  CoefficientOfDynamicFriction=muk  CoefficientOfStaticFriction=mus  NormalDamping=b  NormalDampingUnits=N/(m/s)  NormalStiffness=k  NormalStiffnessUnits=N/m  FrictionalCriticalVelocity=1e-3  FrictionalCriticalVelocityUnits=m/s  ZeroCrossDetectContactStartAndEnd=off  SenseFrictionalForceMagnitude=off  SenseNormalForceMagnitude=off  SenseSeparationDistance=off  NormalTransitionRegionWidth=1e-4  NormalTransitionRegionWidthUnits=m  FrictionType=SmoothStickSlip
      settings: SourceProductName=Multibody
  Spatial Contact Force4 : sm_lib/Forces and Torques/Spatial Contact Force  CoefficientOfDynamicFriction=muk  CoefficientOfStaticFriction=mus  NormalDamping=b  NormalDampingUnits=N/(m/s)  NormalStiffness=k  NormalStiffnessUnits=N/m  FrictionalCriticalVelocity=1e-3  FrictionalCriticalVelocityUnits=m/s  ZeroCrossDetectContactStartAndEnd=on  SenseFrictionalForceMagnitude=off  SenseNormalForceMagnitude=off  SenseSeparationDistance=off  NormalTransitionRegionWidth=1e-5  NormalTransitionRegionWidthUnits=m  FrictionType=SmoothStickSlip
      settings: SourceProductName=Multibody
  Container : PMIOPort  Side=Left
  Part : PMIOPort  Port=2  Side=Right
  connections:
  Spatial Contact Force4/RConn1 -- Spatial Contact Force3/RConn1 -- Part/RConn1 -- Spatial Contact Force2/RConn1 -- Spatial Contact Force1/RConn1 -- Spatial Contact Force7/RConn1
  Simscape Bus/RConn1 -- Container/RConn1
  Simscape Bus/LConn1 -- Spatial Contact Force7/LConn1
  Simscape Bus/LConn2 -- Spatial Contact Force1/LConn1
  Simscape Bus/LConn3 -- Spatial Contact Force2/LConn1
  Simscape Bus/LConn4 -- Spatial Contact Force3/LConn1
  Simscape Bus/LConn5 -- Spatial Contact Force4/LConn1

== system main/Contacts Models Container/Contacts Model-Container5 ==
  Simscape Bus : SimscapeBus  HierarchyStrings=Side1;Side2;Side3;Side4;Bottom
  Spatial Contact Force{1..3,7} (4 alike) : sm_lib/Forces and Torques/Spatial Contact Force  CoefficientOfDynamicFriction=muk  CoefficientOfStaticFriction=mus  NormalDamping=b  NormalDampingUnits=N/(m/s)  NormalStiffness=k  NormalStiffnessUnits=N/m  FrictionalCriticalVelocity=1e-3  FrictionalCriticalVelocityUnits=m/s  ZeroCrossDetectContactStartAndEnd=off  SenseFrictionalForceMagnitude=off  SenseNormalForceMagnitude=off  SenseSeparationDistance=off  NormalTransitionRegionWidth=1e-4  NormalTransitionRegionWidthUnits=m  FrictionType=SmoothStickSlip
      settings: SourceProductName=Multibody
  Spatial Contact Force4 : sm_lib/Forces and Torques/Spatial Contact Force  CoefficientOfDynamicFriction=muk  CoefficientOfStaticFriction=mus  NormalDamping=b  NormalDampingUnits=N/(m/s)  NormalStiffness=k  NormalStiffnessUnits=N/m  FrictionalCriticalVelocity=1e-3  FrictionalCriticalVelocityUnits=m/s  ZeroCrossDetectContactStartAndEnd=on  SenseFrictionalForceMagnitude=off  SenseNormalForceMagnitude=off  SenseSeparationDistance=off  NormalTransitionRegionWidth=1e-5  NormalTransitionRegionWidthUnits=m  FrictionType=SmoothStickSlip
      settings: SourceProductName=Multibody
  Container : PMIOPort  Side=Left
  Part : PMIOPort  Port=2  Side=Right
  connections:
  Spatial Contact Force4/RConn1 -- Spatial Contact Force3/RConn1 -- Part/RConn1 -- Spatial Contact Force2/RConn1 -- Spatial Contact Force1/RConn1 -- Spatial Contact Force7/RConn1
  Simscape Bus/RConn1 -- Container/RConn1
  Simscape Bus/LConn1 -- Spatial Contact Force7/LConn1
  Simscape Bus/LConn2 -- Spatial Contact Force1/LConn1
  Simscape Bus/LConn3 -- Spatial Contact Force2/LConn1
  Simscape Bus/LConn4 -- Spatial Contact Force3/LConn1
  Simscape Bus/LConn5 -- Spatial Contact Force4/LConn1

== system main/End Effector-Part Contact Forces1/End Effector Part 1 ==
  Simscape Bus1 : SimscapeBus  HierarchyStrings=point1;point2;point3
  Spatial Contact Force5 : sm_lib/Forces and Torques/Spatial Contact Force  CoefficientOfDynamicFriction=muk  CoefficientOfStaticFriction=mus  NormalDamping=b  NormalDampingUnits=N/(m/s)  NormalStiffness=k  NormalStiffnessUnits=N/m  FrictionalCriticalVelocity=1e-3  FrictionalCriticalVelocityUnits=m/s  ZeroCrossDetectContactStartAndEnd=off  SenseFrictionalForceMagnitude=off  SenseNormalForceMagnitude=off  SenseSeparationDistance=off  NormalTransitionRegionWidth=1e-4  NormalTransitionRegionWidthUnits=m  FrictionType=SmoothStickSlip
      settings: SourceProductName=Multibody
  Spatial Contact Force6 : sm_lib/Forces and Torques/Spatial Contact Force  CoefficientOfDynamicFriction=muk  CoefficientOfStaticFriction=mus  NormalDamping=b  NormalDampingUnits=N/(m/s)  NormalStiffness=k  NormalStiffnessUnits=N/m  FrictionalCriticalVelocity=1e-3  FrictionalCriticalVelocityUnits=m/s  ZeroCrossDetectContactStartAndEnd=off  SenseFrictionalForceMagnitude=off  SenseNormalForceMagnitude=off  SenseSeparationDistance=off  NormalTransitionRegionWidth=1e-4  NormalTransitionRegionWidthUnits=m  FrictionType=SmoothStickSlip
      settings: SourceProductName=Multibody
  Spatial Contact Force7 : sm_lib/Forces and Torques/Spatial Contact Force  CoefficientOfDynamicFriction=muk  CoefficientOfStaticFriction=mus  NormalDamping=b  NormalDampingUnits=N/(m/s)  NormalStiffness=k  NormalStiffnessUnits=N/m  FrictionalCriticalVelocity=1e-3  FrictionalCriticalVelocityUnits=m/s  ZeroCrossDetectContactStartAndEnd=off  SenseFrictionalForceMagnitude=off  SenseNormalForceMagnitude=off  SenseSeparationDistance=off  NormalTransitionRegionWidth=1e-4  NormalTransitionRegionWidthUnits=m  FrictionType=SmoothStickSlip
      settings: SourceProductName=Multibody
  End Effector : PMIOPort  Side=Left
  Part : PMIOPort  Port=2  Side=Right
  connections:
  Simscape Bus1/LConn1 -- Spatial Contact Force7/LConn1
  Spatial Contact Force5/LConn1 -- Simscape Bus1/LConn3
  Spatial Contact Force6/RConn1 -- Spatial Contact Force5/RConn1 -- Part/RConn1 -- Spatial Contact Force7/RConn1
  Simscape Bus1/LConn2 -- Spatial Contact Force6/LConn1
  Simscape Bus1/RConn1 -- End Effector/RConn1

== system main/End Effector-Part Contact Forces1/End Effector Part 2 ==
  Simscape Bus1 : SimscapeBus  HierarchyStrings=point1;point2;point3
  Spatial Contact Force5 : sm_lib/Forces and Torques/Spatial Contact Force  CoefficientOfDynamicFriction=muk  CoefficientOfStaticFriction=mus  NormalDamping=b  NormalDampingUnits=N/(m/s)  NormalStiffness=k  NormalStiffnessUnits=N/m  FrictionalCriticalVelocity=1e-3  FrictionalCriticalVelocityUnits=m/s  ZeroCrossDetectContactStartAndEnd=off  SenseFrictionalForceMagnitude=off  SenseNormalForceMagnitude=off  SenseSeparationDistance=off  NormalTransitionRegionWidth=1e-4  NormalTransitionRegionWidthUnits=m  FrictionType=SmoothStickSlip
      settings: SourceProductName=Multibody
  Spatial Contact Force6 : sm_lib/Forces and Torques/Spatial Contact Force  CoefficientOfDynamicFriction=muk  CoefficientOfStaticFriction=mus  NormalDamping=b  NormalDampingUnits=N/(m/s)  NormalStiffness=k  NormalStiffnessUnits=N/m  FrictionalCriticalVelocity=1e-3  FrictionalCriticalVelocityUnits=m/s  ZeroCrossDetectContactStartAndEnd=off  SenseFrictionalForceMagnitude=off  SenseNormalForceMagnitude=off  SenseSeparationDistance=off  NormalTransitionRegionWidth=1e-4  NormalTransitionRegionWidthUnits=m  FrictionType=SmoothStickSlip
      settings: SourceProductName=Multibody
  Spatial Contact Force7 : sm_lib/Forces and Torques/Spatial Contact Force  CoefficientOfDynamicFriction=muk  CoefficientOfStaticFriction=mus  NormalDamping=b  NormalDampingUnits=N/(m/s)  NormalStiffness=k  NormalStiffnessUnits=N/m  FrictionalCriticalVelocity=1e-3  FrictionalCriticalVelocityUnits=m/s  ZeroCrossDetectContactStartAndEnd=off  SenseFrictionalForceMagnitude=off  SenseNormalForceMagnitude=off  SenseSeparationDistance=off  NormalTransitionRegionWidth=1e-4  NormalTransitionRegionWidthUnits=m  FrictionType=SmoothStickSlip
      settings: SourceProductName=Multibody
  End Effector : PMIOPort  Side=Left
  Part : PMIOPort  Port=2  Side=Right
  connections:
  Simscape Bus1/LConn1 -- Spatial Contact Force7/LConn1
  Spatial Contact Force5/LConn1 -- Simscape Bus1/LConn3
  Spatial Contact Force6/RConn1 -- Spatial Contact Force5/RConn1 -- Part/RConn1 -- Spatial Contact Force7/RConn1
  Simscape Bus1/LConn2 -- Spatial Contact Force6/LConn1
  Simscape Bus1/RConn1 -- End Effector/RConn1

== system main/End Effector-Part Contact Forces1/End Effector Part 3 ==
  Simscape Bus1 : SimscapeBus  HierarchyStrings=point1;point2;point3
  Spatial Contact Force5 : sm_lib/Forces and Torques/Spatial Contact Force  CoefficientOfDynamicFriction=muk  CoefficientOfStaticFriction=mus  NormalDamping=b  NormalDampingUnits=N/(m/s)  NormalStiffness=k  NormalStiffnessUnits=N/m  FrictionalCriticalVelocity=1e-3  FrictionalCriticalVelocityUnits=m/s  ZeroCrossDetectContactStartAndEnd=off  SenseFrictionalForceMagnitude=off  SenseNormalForceMagnitude=off  SenseSeparationDistance=off  NormalTransitionRegionWidth=1e-4  NormalTransitionRegionWidthUnits=m  FrictionType=SmoothStickSlip
      settings: SourceProductName=Multibody
  Spatial Contact Force6 : sm_lib/Forces and Torques/Spatial Contact Force  CoefficientOfDynamicFriction=muk  CoefficientOfStaticFriction=mus  NormalDamping=b  NormalDampingUnits=N/(m/s)  NormalStiffness=k  NormalStiffnessUnits=N/m  FrictionalCriticalVelocity=1e-3  FrictionalCriticalVelocityUnits=m/s  ZeroCrossDetectContactStartAndEnd=off  SenseFrictionalForceMagnitude=off  SenseNormalForceMagnitude=off  SenseSeparationDistance=off  NormalTransitionRegionWidth=1e-4  NormalTransitionRegionWidthUnits=m  FrictionType=SmoothStickSlip
      settings: SourceProductName=Multibody
  Spatial Contact Force7 : sm_lib/Forces and Torques/Spatial Contact Force  CoefficientOfDynamicFriction=muk  CoefficientOfStaticFriction=mus  NormalDamping=b  NormalDampingUnits=N/(m/s)  NormalStiffness=k  NormalStiffnessUnits=N/m  FrictionalCriticalVelocity=1e-3  FrictionalCriticalVelocityUnits=m/s  ZeroCrossDetectContactStartAndEnd=off  SenseFrictionalForceMagnitude=off  SenseNormalForceMagnitude=off  SenseSeparationDistance=off  NormalTransitionRegionWidth=1e-4  NormalTransitionRegionWidthUnits=m  FrictionType=SmoothStickSlip
      settings: SourceProductName=Multibody
  End Effector : PMIOPort  Side=Left
  Part : PMIOPort  Port=2  Side=Right
  connections:
  Simscape Bus1/LConn1 -- Spatial Contact Force7/LConn1
  Spatial Contact Force5/LConn1 -- Simscape Bus1/LConn3
  Spatial Contact Force6/RConn1 -- Spatial Contact Force5/RConn1 -- Part/RConn1 -- Spatial Contact Force7/RConn1
  Simscape Bus1/LConn2 -- Spatial Contact Force6/LConn1
  Simscape Bus1/RConn1 -- End Effector/RConn1

== system main/End Effector-Part Contact Forces1/End Effector Part 4 ==
  Simscape Bus1 : SimscapeBus  HierarchyStrings=point1;point2;point3
  Spatial Contact Force5 : sm_lib/Forces and Torques/Spatial Contact Force  CoefficientOfDynamicFriction=muk  CoefficientOfStaticFriction=mus  NormalDamping=b  NormalDampingUnits=N/(m/s)  NormalStiffness=k  NormalStiffnessUnits=N/m  FrictionalCriticalVelocity=1e-3  FrictionalCriticalVelocityUnits=m/s  ZeroCrossDetectContactStartAndEnd=off  SenseFrictionalForceMagnitude=off  SenseNormalForceMagnitude=off  SenseSeparationDistance=off  NormalTransitionRegionWidth=1e-4  NormalTransitionRegionWidthUnits=m  FrictionType=SmoothStickSlip
      settings: SourceProductName=Multibody
  Spatial Contact Force6 : sm_lib/Forces and Torques/Spatial Contact Force  CoefficientOfDynamicFriction=muk  CoefficientOfStaticFriction=mus  NormalDamping=b  NormalDampingUnits=N/(m/s)  NormalStiffness=k  NormalStiffnessUnits=N/m  FrictionalCriticalVelocity=1e-3  FrictionalCriticalVelocityUnits=m/s  ZeroCrossDetectContactStartAndEnd=off  SenseFrictionalForceMagnitude=off  SenseNormalForceMagnitude=off  SenseSeparationDistance=off  NormalTransitionRegionWidth=1e-4  NormalTransitionRegionWidthUnits=m  FrictionType=SmoothStickSlip
      settings: SourceProductName=Multibody
  Spatial Contact Force7 : sm_lib/Forces and Torques/Spatial Contact Force  CoefficientOfDynamicFriction=muk  CoefficientOfStaticFriction=mus  NormalDamping=b  NormalDampingUnits=N/(m/s)  NormalStiffness=k  NormalStiffnessUnits=N/m  FrictionalCriticalVelocity=1e-3  FrictionalCriticalVelocityUnits=m/s  ZeroCrossDetectContactStartAndEnd=off  SenseFrictionalForceMagnitude=off  SenseNormalForceMagnitude=off  SenseSeparationDistance=off  NormalTransitionRegionWidth=1e-4  NormalTransitionRegionWidthUnits=m  FrictionType=SmoothStickSlip
      settings: SourceProductName=Multibody
  End Effector : PMIOPort  Side=Left
  Part : PMIOPort  Port=2  Side=Right
  connections:
  Simscape Bus1/LConn1 -- Spatial Contact Force7/LConn1
  Spatial Contact Force5/LConn1 -- Simscape Bus1/LConn3
  Spatial Contact Force6/RConn1 -- Spatial Contact Force5/RConn1 -- Part/RConn1 -- Spatial Contact Force7/RConn1
  Simscape Bus1/LConn2 -- Spatial Contact Force6/LConn1
  Simscape Bus1/RConn1 -- End Effector/RConn1

== system main/End Effector-Part Contact Forces1/End Effector Part 5 ==
  Simscape Bus1 : SimscapeBus  HierarchyStrings=point1;point2;point3
  Spatial Contact Force5 : sm_lib/Forces and Torques/Spatial Contact Force  CoefficientOfDynamicFriction=muk  CoefficientOfStaticFriction=mus  NormalDamping=b  NormalDampingUnits=N/(m/s)  NormalStiffness=k  NormalStiffnessUnits=N/m  FrictionalCriticalVelocity=1e-3  FrictionalCriticalVelocityUnits=m/s  ZeroCrossDetectContactStartAndEnd=off  SenseFrictionalForceMagnitude=off  SenseNormalForceMagnitude=off  SenseSeparationDistance=off  NormalTransitionRegionWidth=1e-4  NormalTransitionRegionWidthUnits=m  FrictionType=SmoothStickSlip
      settings: SourceProductName=Multibody
  Spatial Contact Force6 : sm_lib/Forces and Torques/Spatial Contact Force  CoefficientOfDynamicFriction=muk  CoefficientOfStaticFriction=mus  NormalDamping=b  NormalDampingUnits=N/(m/s)  NormalStiffness=k  NormalStiffnessUnits=N/m  FrictionalCriticalVelocity=1e-3  FrictionalCriticalVelocityUnits=m/s  ZeroCrossDetectContactStartAndEnd=off  SenseFrictionalForceMagnitude=off  SenseNormalForceMagnitude=off  SenseSeparationDistance=off  NormalTransitionRegionWidth=1e-4  NormalTransitionRegionWidthUnits=m  FrictionType=SmoothStickSlip
      settings: SourceProductName=Multibody
  Spatial Contact Force7 : sm_lib/Forces and Torques/Spatial Contact Force  CoefficientOfDynamicFriction=muk  CoefficientOfStaticFriction=mus  NormalDamping=b  NormalDampingUnits=N/(m/s)  NormalStiffness=k  NormalStiffnessUnits=N/m  FrictionalCriticalVelocity=1e-3  FrictionalCriticalVelocityUnits=m/s  ZeroCrossDetectContactStartAndEnd=off  SenseFrictionalForceMagnitude=off  SenseNormalForceMagnitude=off  SenseSeparationDistance=off  NormalTransitionRegionWidth=1e-4  NormalTransitionRegionWidthUnits=m  FrictionType=SmoothStickSlip
      settings: SourceProductName=Multibody
  End Effector : PMIOPort  Side=Left
  Part : PMIOPort  Port=2  Side=Right
  connections:
  Simscape Bus1/LConn1 -- Spatial Contact Force7/LConn1
  Spatial Contact Force5/LConn1 -- Simscape Bus1/LConn3
  Spatial Contact Force6/RConn1 -- Spatial Contact Force5/RConn1 -- Part/RConn1 -- Spatial Contact Force7/RConn1
  Simscape Bus1/LConn2 -- Spatial Contact Force6/LConn1
  Simscape Bus1/RConn1 -- End Effector/RConn1
